simulink model "machinelab"  (R2019b)
settings: Solver=FixedStepAuto  StartTime=0.0  StopTime=0.5  FixedStep=0.00001  MaxStep=0.0005  RelTol=1e-3
model workspace (MAT data in the model file):
  t = 5
  torque_in = 0
values from neighbouring files (symbols this model uses):
  J = 0.22    [lab4.m]
  La = (5+(N/2000))/1e3    (= 0.0092985)    [lab4.m]
  Lf = (5+(N/1e3))    (= 13.597)    [lab4.m]
  N = 8597    [lab4.m]
  Ra = (0.2+(N/12e3))    (= 0.916416666667)    [lab4.m]
  Rf = (40+(N/100))    (= 125.97)    [lab4.m]
libraries: powerlib x6
settings Model: Creator=100448597  LastModifiedBy=robom
settings DataIOCC: SaveOutput=off  InspectSignalLogs=on  ReturnWorkspaceOutputs=off
settings DebuggingCC: ArithmeticOperatorsInVariantConditions=warning
settings SFSimCC: SimUseLocalCustomCode=off  CustomCodeUndefinedFunction=UseInterfaceOnly
settings RTWCC: RTWUseLocalCustomCode=off

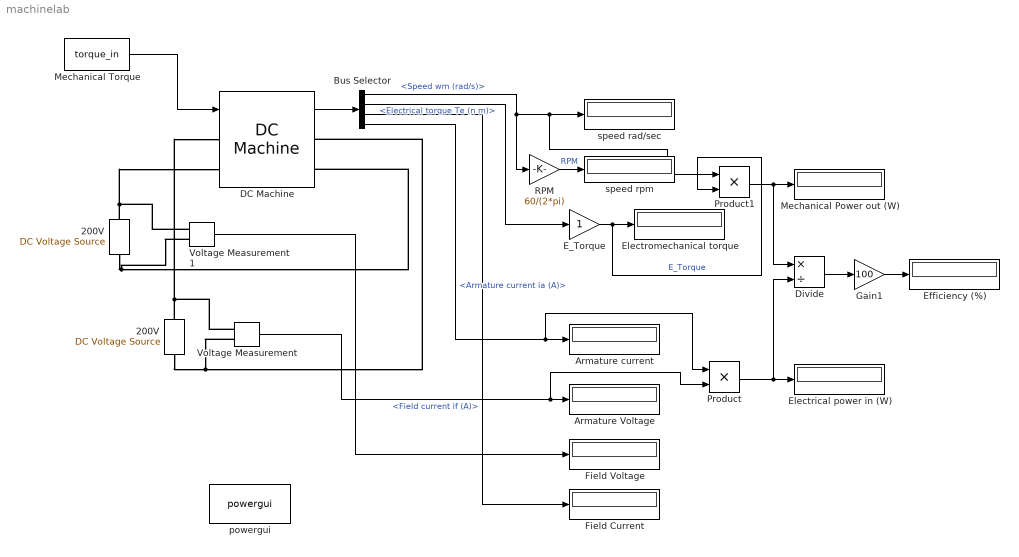
== system machinelab ==
  " 200V" : powerlib/Electrical Sources/DC Voltage Source  Amplitude=200  Measurements=None
      settings: SourceProductName=Simscape Electrical
  200V : powerlib/Electrical Sources/DC Voltage Source  Amplitude=200  Measurements=None
      settings: SourceProductName=Simscape Electrical
  "Armature Voltage " : Display
  "Armature current " : Display
  Bus Selector : BusSelector  OutputSignals=Speed wm (rad/s),Electrical torque Te (n m),Field current if (A),Armature current ia (A)
  DC Machine : powerlib/Machines/DC Machine  PresetModel=No  MechanicalLoad=Torque TL  FieldType=Wound  ShowDetailedParameters=on  MeasurementBus=off  RLa="[ Ra  La]"  RLf="[ Rf  Lf]"  Laf=Laf  MachineConstant=Torque constant (N.m/A)  Ke=1.8  Kt=1.8  J=J  Bm=B  Tf=Tf  w0=0  Ifinit=0  TsPowergui=0  TsBlock=-1
      settings: SourceProductName=Simscape Electrical
  Divide : Product  Inputs=*/
  E_Torque : Gain
  Efficiency (%) : Display
  Electrical power in (W) : Display
  Electromechanical torque : Display
  Field Current : Display
  Field Voltage : Display
  Gain1 : Gain  Gain=100
  Mechanical Power out (W) : Display
  Mechanical Torque : Constant  Value=torque_in
  Product : Product
  Product1 : Product
  RPM : Gain  Gain=60/(2*pi)
  Voltage Measurement : powerlib/Measurements/Voltage Measurement  PhasorSimulation=off  OutputType=Complex  PSBequivalent=0
      settings: SourceProductName=Simscape Electrical
  Voltage Measurement1 : powerlib/Measurements/Voltage Measurement  PhasorSimulation=off  OutputType=Complex  PSBequivalent=0
      settings: SourceProductName=Simscape Electrical
  powergui : powerlib/powergui  Priority=1  SimulationMode=Continuous  SampleTime=50e-6  frequency=60  Iterations=50  frequencyindice=0  Pbase=100e6  ErrMax=1e-4  UnitsV=kV  UnitsW=MW  buscounter=0  FunctionMessages=off  echomessages=off  EnableUseOfTLC=off  CurrentSourceSwitches=off  DisableSnubberDevices=off  DisableRonSwitches=off  DisableVfSwitches=off  DisplayEquations=off  AutomaticDiscreteSolvers=off  SolverType=Tustin/Backward Euler (TBE)  Interpol=off  ExternalGateDelay=off  methode=off  Ts=100  x0status=blocks  SPID=off  SwTol=0  HookPort=off  NonlinearTolerance=1e-4  nMaxIteration=100  ContinueOnMaxIteration=off  RestoreLinks=warning  ResistiveCurrentMeasurement=off  Frange=[0:2:500]  Ylog=off  Xlog=on  ShowGrid=off  save=off  variable=ZData  structure=0  ZoomFFT=off  StartTime=0.0  cycles=1  DisplayStyle=1  fundamental=60  FreqAxis=off  MaxFrequency=1000  frequencyindicesteady=1  RmsSteady=1  display=off
      settings: SourceProductName=Simscape Electrical
  speed rad/sec : Display
  "speed rpm " : Display
  wires:
  DC Machine/1 -> Bus Selector/1
  Bus Selector/2 -> E_Torque/1  "<Electrical torque Te (n m)>"
  Bus Selector/1 -> RPM/1, Product1/1, speed rad/sec/1  "<Speed wm (rad/s)>"
  Bus Selector/3 -> Field Current/1  "<Field current if (A)>"
  Bus Selector/4 -> Product/1, "Armature current "/1  "<Armature current ia (A)>"
  Voltage Measurement/1 -> Product/2, "Armature Voltage "/1
  Voltage Measurement1/1 -> Field Voltage/1
  Product/1 -> Divide/2, Electrical power in (W)/1
  Product1/1 -> Divide/1, Mechanical Power out (W)/1
  Divide/1 -> Gain1/1
  Gain1/1 -> Efficiency (%)/1
  Mechanical Torque/1 -> DC Machine/1
  RPM/1 -> "speed rpm "/1  "RPM"
  E_Torque/1 -> Product1/2, Electromechanical torque/1  "E_Torque"
  connections:
  " 200V"/LConn1 -- Voltage Measurement1/LConn2 -- DC Machine/RConn2
  200V/LConn1 -- Voltage Measurement/LConn2 -- DC Machine/RConn1
  200V/RConn1 -- DC Machine/LConn1 -- Voltage Measurement/LConn1
  " 200V"/RConn1 -- Voltage Measurement1/LConn1 -- DC Machine/LConn2
